simulink model "EECS_419_Homework_4_Speed"  (R2025a)
settings: Solver=VariableStepAuto  StartTime=0.0  StopTime=10.0  RelTol=1e-3
undefined symbols (not defined in the file or in its folder): b_r, H
libraries: slpidlib x3
settings Model: Creator=petercauchy  LastModifiedBy=petercauchy

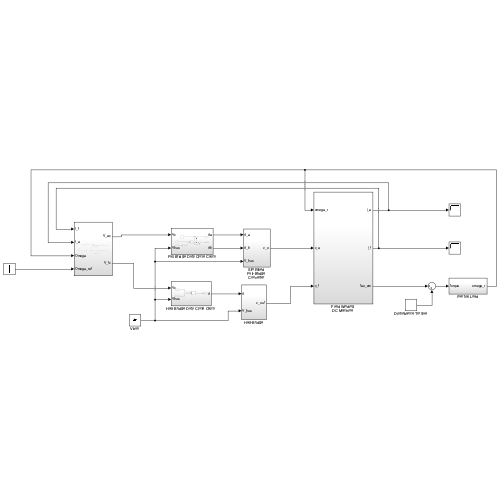
[thumbnail: Simulink's stored preview of the top-level diagram]
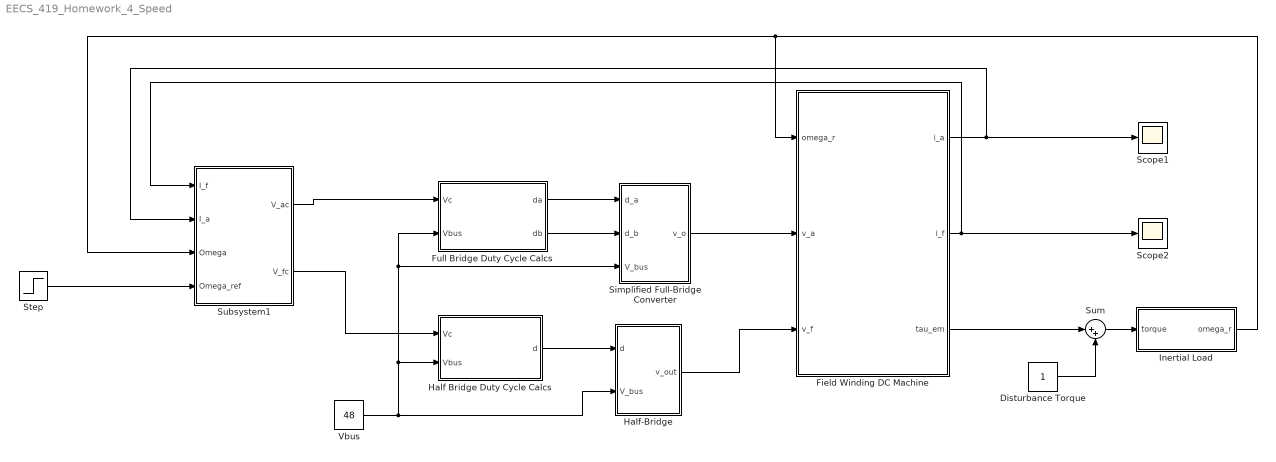
== system EECS_419_Homework_4_Speed ==
  Disturbance Torque : Constant
  Field Winding DC Machine : Subsystem
  Full Bridge Duty Cycle Calcs : Subsystem
  Half Bridge Duty Cycle Calcs : Subsystem
  Half-Bridge : Subsystem
  Inertial Load : Subsystem
  Scope1 : Scope
      settings: ActiveDisplayYMinimum=-27.326179749538095  ActiveDisplayYMaximum=3.1844313093536782
  Scope2 : Scope
      settings: ActiveDisplayYMinimum=-0.0328865701172645  ActiveDisplayYMaximum=0.29597913105538054  DataLoggingVariableName=ScopeData2
  Simplified Full-Bridge Converter : Subsystem
  Step : Step  After=5  SampleTime=0
  Subsystem1 : Subsystem
  Sum : Sum  Inputs=|++
  Vbus : Constant  Value=48
  wires:
  Subsystem1/1(V_ac) -> Full Bridge Duty Cycle Calcs/1(Vc)
  Field Winding DC Machine/3(tau_em) -> Sum/1
  Field Winding DC Machine/1(i_a) -> Scope1/1, Subsystem1/2(I_a)
  Subsystem1/2(V_fc) -> Half Bridge Duty Cycle Calcs/1(Vc)
  Vbus/1 -> Half-Bridge/2(V_bus), Half Bridge Duty Cycle Calcs/2(Vbus), Simplified Full-Bridge Converter/3(V_bus), Full Bridge Duty Cycle Calcs/2(Vbus)
  Half Bridge Duty Cycle Calcs/1(d) -> Half-Bridge/1(d)
  Full Bridge Duty Cycle Calcs/2(db) -> Simplified Full-Bridge Converter/2(d_b)
  Field Winding DC Machine/2(i_f) -> Scope2/1, Subsystem1/1(I_f)
  Full Bridge Duty Cycle Calcs/1(da) -> Simplified Full-Bridge Converter/1(d_a)
  Half-Bridge/1(v_out) -> Field Winding DC Machine/3(v_f)
  Simplified Full-Bridge Converter/1(v_o) -> Field Winding DC Machine/2(v_a)
  Disturbance Torque/1 -> Sum/2
  Sum/1 -> Inertial Load/1(torque)
  Inertial Load/1(omega_r) -> Field Winding DC Machine/1(omega_r), Subsystem1/3(Omega)
  Step/1 -> Subsystem1/4(Omega_ref)

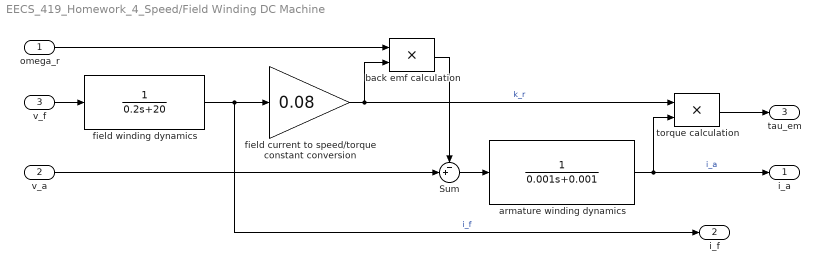
== system EECS_419_Homework_4_Speed/Field Winding DC Machine ==
  omega_r : Inport
  v_a : Inport  Port=2
  v_f : Inport  Port=3
  Sum : Sum  Inputs=-+|  SaturateOnIntegerOverflow=on
  armature winding dynamics : TransferFcn  Denominator=[0.001 0.001]
  back emf calculation : Product  SaturateOnIntegerOverflow=on  OutDataTypeStr=Inherit: Same as first input
  field current to speed/torque constant conversion : Gain  Gain=0.08  SaturateOnIntegerOverflow=on  OutDataTypeStr=Inherit: Same as input  ParamDataTypeStr=Inherit: Same as input
  field winding dynamics : TransferFcn  Denominator=[0.2 20]
  torque calculation : Product  SaturateOnIntegerOverflow=on  OutDataTypeStr=Inherit: Same as first input
  i_a : Outport
  i_f : Outport  Port=2
  tau_em : Outport  Port=3
  wires:
  back emf calculation/1 -> Sum/1
  v_a/1 -> Sum/2
  Sum/1 -> armature winding dynamics/1
  armature winding dynamics/1 -> i_a/1, torque calculation/2  "i_a"
  v_f/1 -> field winding dynamics/1
  field winding dynamics/1 -> i_f/1, field current to speed/torque constant conversion/1  "i_f"
  field current to speed/torque constant conversion/1 -> back emf calculation/2, torque calculation/1  "k_r"
  omega_r/1 -> back emf calculation/1
  torque calculation/1 -> tau_em/1

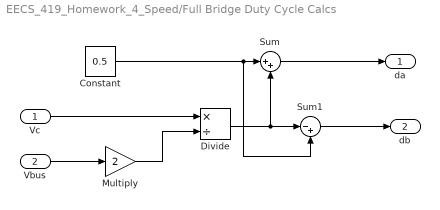
== system EECS_419_Homework_4_Speed/Full Bridge Duty Cycle Calcs ==
  Vc : Inport
  Vbus : Inport  Port=2
  Constant : Constant  Value=0.5
  Divide : Product  Inputs=*/
  Multiply : Gain  Gain=2
  Sum : Sum  Inputs=|++
  Sum1 : Sum  Inputs=|-+
  da : Outport
  db : Outport  Port=2
  wires:
  Vc/1 -> Divide/1
  Vbus/1 -> Multiply/1
  Constant/1 -> Sum1/2, Sum/1
  Sum/1 -> da/1
  Divide/1 -> Sum1/1, Sum/2
  Multiply/1 -> Divide/2
  Sum1/1 -> db/1

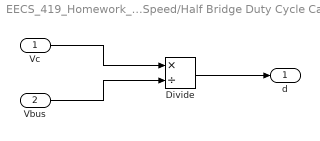
== system EECS_419_Homework_4_Speed/Half Bridge Duty Cycle Calcs ==
  Vc : Inport
  Vbus : Inport  Port=2
  Divide : Product  Inputs=*/
  d : Outport
  wires:
  Vbus/1 -> Divide/2
  Vc/1 -> Divide/1
  Divide/1 -> d/1

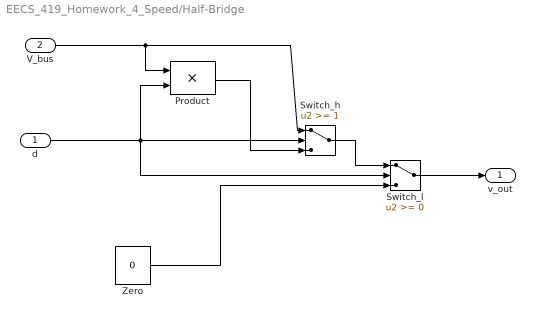
== system EECS_419_Homework_4_Speed/Half-Bridge ==
  d : Inport
  V_bus : Inport  Port=2
  Product : Product  SaturateOnIntegerOverflow=on  OutDataTypeStr=Inherit: Same as first input
  Switch_h : Switch  Threshold=1  InputSameDT=off
  Switch_l : Switch  InputSameDT=off
  Zero : Constant  Value=0
  v_out : Outport  VectorParamsAs1DForOutWhenUnconnected=off
  wires:
  d/1 -> Switch_h/2, Product/2, Switch_l/2
  V_bus/1 -> Switch_h/1, Product/1
  Product/1 -> Switch_h/3
  Zero/1 -> Switch_l/3
  Switch_h/1 -> Switch_l/1
  Switch_l/1 -> v_out/1

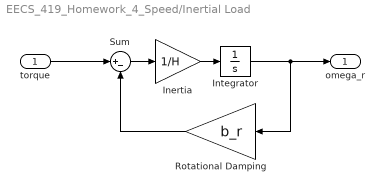
== system EECS_419_Homework_4_Speed/Inertial Load ==
  torque : Inport
  Inertia : Gain  Gain=1/H  SaturateOnIntegerOverflow=on  OutDataTypeStr=Inherit: Same as input  ParamDataTypeStr=Inherit: Same as input
  Integrator : Integrator
  Rotational Damping : Gain  Gain=b_r  SaturateOnIntegerOverflow=on  OutDataTypeStr=Inherit: Same as input  ParamDataTypeStr=Inherit: Same as input
  Sum : Sum  Inputs=|+-  SaturateOnIntegerOverflow=on
  omega_r : Outport
  wires:
  Integrator/1 -> omega_r/1, Rotational Damping/1
  torque/1 -> Sum/1
  Sum/1 -> Inertia/1
  Inertia/1 -> Integrator/1
  Rotational Damping/1 -> Sum/2

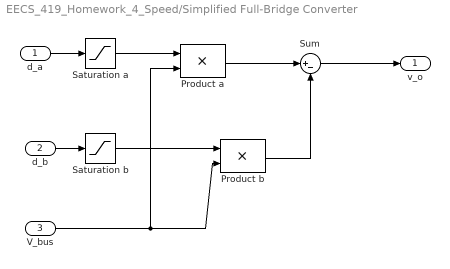
== system EECS_419_Homework_4_Speed/Simplified Full-Bridge Converter ==
  d_a : Inport
  d_b : Inport  Port=2
  V_bus : Inport  Port=3
  Product a : Product  SaturateOnIntegerOverflow=on  OutDataTypeStr=Inherit: Same as first input
  Product b : Product  SaturateOnIntegerOverflow=on  OutDataTypeStr=Inherit: Same as first input
  Saturation a : Saturate  UpperLimit=1  LowerLimit=0
  Saturation b : Saturate  UpperLimit=1  LowerLimit=0
  Sum : Sum  Inputs=|+-  SaturateOnIntegerOverflow=on
  v_o : Outport  VectorParamsAs1DForOutWhenUnconnected=off
  wires:
  d_a/1 -> Saturation a/1
  d_b/1 -> Saturation b/1
  Product a/1 -> Sum/1
  Product b/1 -> Sum/2
  Sum/1 -> v_o/1
  Saturation a/1 -> Product a/1
  V_bus/1 -> Product a/2, Product b/2
  Saturation b/1 -> Product b/1

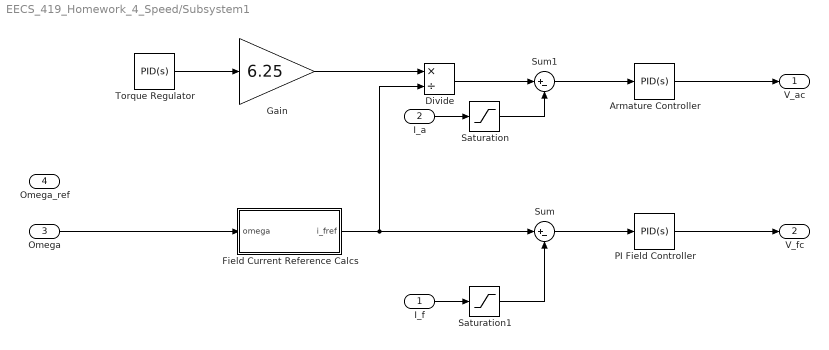
== system EECS_419_Homework_4_Speed/Subsystem1 ==
  I_f : Inport
  I_a : Inport  Port=2
  Omega : Inport  Port=3
  Omega_ref : Inport  Port=4
  Armature Controller : slpidlib/PID Controller  Controller=PID  Form=Parallel  TimeDomain=Continuous-time  UseExternalTs=off  SampleTime=-1  IntegratorMethod=Forward Euler  FilterMethod=Forward Euler  ControllerParametersSource=internal  P=6.28  I=6.28  UseKiTs=off  D=0  UseExternalDerivativeSource=off  N=1  UseFilter=on  TunerSelectOption=Transfer Function Based (PID Tuner App)  InitialConditionSource=internal  InitialConditionForIntegrator=0  InitialConditionForFilter=0  DifferentiatorICPrevScaledInput=0  ExternalReset=none  TrackingMode=off  Kt=1  LimitOutput=on  SatLimitsSource=internal  UpperSaturationLimit=48  LowerSaturationLimit=-48  LinearizeAsGain=on  AntiWindupMode=none  Kb=1  LimitIntegrator=off  UpperIntegratorSaturationLimit=inf  LowerIntegratorSaturationLimit=-inf  POutMin=[]  POutMax=[]  IOutMin=[]  IOutMax=[]  DOutMin=[]  DOutMax=[]  NOutMin=[]  NOutMax=[]  SumOutMin=[]  SumOutMax=[]  SaturationOutMin=[]  SaturationOutMax=[]  PParamMin=[]  PParamMax=[]  IParamMin=[]  IParamMax=[]  DParamMin=[]  DParamMax=[]  NParamMin=[]  NParamMax=[]  KbParamMin=[]  KbParamMax=[]  KtParamMin=[]  KtParamMax=[]  KbOutMin=[]  KbOutMax=[]  KtOutMin=[]  KtOutMax=[]  IntegratorOutMin=[]  IntegratorOutMax=[]  FilterOutMin=[]  FilterOutMax=[]  SumI1OutMin=[]  SumI1OutMax=[]  SumI2OutMin=[]  SumI2OutMax=[]  SumI3OutMin=[]  SumI3OutMax=[]  SumI4OutMin=[]  SumI4OutMax=[]  SumDOutMin=[]  SumDOutMax=[]  DifferentiatorOutMin=[]  DifferentiatorOutMax=[]  FilterDiffOutCoefMin=[]  FilterDiffOutCoefMax=[]  ReciprocalOutMin=[]  ReciprocalOutMax=[]  SumDenOutMin=[]  SumDenOutMax=[]  SumNumOutMin=[]  SumNumOutMax=[]  DivideOutMin=[]  DivideOutMax=[]  UdiffTsProdOutMin=[]  UdiffTsProdOutMax=[]  NTsProdOutMin=[]  NTsProdOutMax=[]  UintegralTsProdOutMin=[]  UintegralTsProdOutMax=[]  UngainTsProdOutMin=[]  UngainTsProdOutMax=[]  ClampingZeroOutDataTypeStr=Inherit: Inherit via back propagation  ClampingZeroOutMin=[]  ClampingZeroOutMax=[]  FilterDenConstantOutDataTypeStr=Inherit: Inherit via back propagation  FilterDenConstantOutMin=[]  FilterDenConstantOutMax=[]  PCopyOutDataTypeStr=Inherit: Inherit via back propagation  PCopyOutMin=[]  PCopyOutMax=[]  NCopyOutDataTypeStr=Inherit: Inherit via back propagation  NCopyOutMin=[]  NCopyOutMax=[]  IntegratorContinuousStateAttributes=''  IntegratorStateMustResolveToSignalObject=off  IntegratorRTWStateStorageClass=Auto  FilterContinuousStateAttributes=''  FilterStateMustResolveToSignalObject=off  FilterRTWStateStorageClass=Auto  ParallelPVariant=InternalParameters  IdealPVariant=Disabled  IVariant=InternalParameters  DVariant=InternalParameters  IntegratorVariant=Continuous  SatVariant=Enabled  AWVariant=Passthrough  PCopyVariant=Disabled  TRVariant=Disabled  FdbkBlocksVariant=Forward  IdealPFdbkVariant=Disabled  SatFdbkVariant=Disabled  DerivativeFilterVariant=ContFilter  NVariant=InternalParameters  NCopyVariant=Disabled  FilterICVariant=InternalICsFilter  IntegratorICVariant=InternalICs  ExternalResetVariant=Disabled  TRSumVariant=Passthrough  SumFdbkVariant=Disabled  SumVariant=Sum_PID  TsampFilterVariant=InternalTs  TsampNgainVariant=Passthrough  TsampIntegralVariant=Disabled_SignalSpec  ExternalSaturationOutDataTypeStr=Inherit: Same as second input  DerivativeSourceVariant=ErrorSignal  PreIntVariant=InternalPreInt
  Divide : Product  Inputs=*/
  Field Current Reference Calcs : Subsystem
  Gain : Gain  Gain=6.25
  PI Field Controller : slpidlib/PID Controller  Controller=PID  Form=Parallel  TimeDomain=Continuous-time  UseExternalTs=off  SampleTime=-1  IntegratorMethod=Forward Euler  FilterMethod=Forward Euler  ControllerParametersSource=internal  P=1256.6  I=1.256e6  UseKiTs=off  D=0  UseExternalDerivativeSource=off  N=1  UseFilter=on  TunerSelectOption=Transfer Function Based (PID Tuner App)  InitialConditionSource=internal  InitialConditionForIntegrator=0  InitialConditionForFilter=0  DifferentiatorICPrevScaledInput=0  ExternalReset=none  TrackingMode=off  Kt=1  LimitOutput=on  SatLimitsSource=internal  UpperSaturationLimit=48  LowerSaturationLimit=0  LinearizeAsGain=on  AntiWindupMode=none  Kb=1  LimitIntegrator=off  UpperIntegratorSaturationLimit=inf  LowerIntegratorSaturationLimit=-inf  POutMin=[]  POutMax=[]  IOutMin=[]  IOutMax=[]  DOutMin=[]  DOutMax=[]  NOutMin=[]  NOutMax=[]  SumOutMin=[]  SumOutMax=[]  SaturationOutMin=[]  SaturationOutMax=[]  PParamMin=[]  PParamMax=[]  IParamMin=[]  IParamMax=[]  DParamMin=[]  DParamMax=[]  NParamMin=[]  NParamMax=[]  KbParamMin=[]  KbParamMax=[]  KtParamMin=[]  KtParamMax=[]  KbOutMin=[]  KbOutMax=[]  KtOutMin=[]  KtOutMax=[]  IntegratorOutMin=[]  IntegratorOutMax=[]  FilterOutMin=[]  FilterOutMax=[]  SumI1OutMin=[]  SumI1OutMax=[]  SumI2OutMin=[]  SumI2OutMax=[]  SumI3OutMin=[]  SumI3OutMax=[]  SumI4OutMin=[]  SumI4OutMax=[]  SumDOutMin=[]  SumDOutMax=[]  DifferentiatorOutMin=[]  DifferentiatorOutMax=[]  FilterDiffOutCoefMin=[]  FilterDiffOutCoefMax=[]  ReciprocalOutMin=[]  ReciprocalOutMax=[]  SumDenOutMin=[]  SumDenOutMax=[]  SumNumOutMin=[]  SumNumOutMax=[]  DivideOutMin=[]  DivideOutMax=[]  UdiffTsProdOutMin=[]  UdiffTsProdOutMax=[]  NTsProdOutMin=[]  NTsProdOutMax=[]  UintegralTsProdOutMin=[]  UintegralTsProdOutMax=[]  UngainTsProdOutMin=[]  UngainTsProdOutMax=[]  ClampingZeroOutDataTypeStr=Inherit: Inherit via back propagation  ClampingZeroOutMin=[]  ClampingZeroOutMax=[]  FilterDenConstantOutDataTypeStr=Inherit: Inherit via back propagation  FilterDenConstantOutMin=[]  FilterDenConstantOutMax=[]  PCopyOutDataTypeStr=Inherit: Inherit via back propagation  PCopyOutMin=[]  PCopyOutMax=[]  NCopyOutDataTypeStr=Inherit: Inherit via back propagation  NCopyOutMin=[]  NCopyOutMax=[]  IntegratorContinuousStateAttributes=''  IntegratorStateMustResolveToSignalObject=off  IntegratorRTWStateStorageClass=Auto  FilterContinuousStateAttributes=''  FilterStateMustResolveToSignalObject=off  FilterRTWStateStorageClass=Auto  ParallelPVariant=InternalParameters  IdealPVariant=Disabled  IVariant=InternalParameters  DVariant=InternalParameters  IntegratorVariant=Continuous  SatVariant=Enabled  AWVariant=Passthrough  PCopyVariant=Disabled  TRVariant=Disabled  FdbkBlocksVariant=Forward  IdealPFdbkVariant=Disabled  SatFdbkVariant=Disabled  DerivativeFilterVariant=ContFilter  NVariant=InternalParameters  NCopyVariant=Disabled  FilterICVariant=InternalICsFilter  IntegratorICVariant=InternalICs  ExternalResetVariant=Disabled  TRSumVariant=Passthrough  SumFdbkVariant=Disabled  SumVariant=Sum_PID  TsampFilterVariant=InternalTs  TsampNgainVariant=Passthrough  TsampIntegralVariant=Disabled_SignalSpec  ExternalSaturationOutDataTypeStr=Inherit: Same as second input  DerivativeSourceVariant=ErrorSignal  PreIntVariant=InternalPreInt
  Saturation : Saturate  UpperLimit=100  LowerLimit=-100
  Saturation1 : Saturate  UpperLimit=1  LowerLimit=-1
  Sum : Sum  Inputs=|+-
  Sum1 : Sum  Inputs=|+-
  Torque Regulator : slpidlib/PID Controller  Controller=PID  Form=Parallel  TimeDomain=Continuous-time  UseExternalTs=off  SampleTime=-1  IntegratorMethod=Forward Euler  FilterMethod=Forward Euler  ControllerParametersSource=internal  P=78.5  I=78.5  UseKiTs=off  D=0  UseExternalDerivativeSource=off  N=1  UseFilter=on  TunerSelectOption=Transfer Function Based (PID Tuner App)  InitialConditionSource=internal  InitialConditionForIntegrator=0  InitialConditionForFilter=0  DifferentiatorICPrevScaledInput=0  ExternalReset=none  TrackingMode=off  Kt=1  LimitOutput=off  SatLimitsSource=internal  UpperSaturationLimit=inf  LowerSaturationLimit=-inf  LinearizeAsGain=on  AntiWindupMode=none  Kb=1  LimitIntegrator=off  UpperIntegratorSaturationLimit=inf  LowerIntegratorSaturationLimit=-inf  POutMin=[]  POutMax=[]  IOutMin=[]  IOutMax=[]  DOutMin=[]  DOutMax=[]  NOutMin=[]  NOutMax=[]  SumOutMin=[]  SumOutMax=[]  SaturationOutMin=[]  SaturationOutMax=[]  PParamMin=[]  PParamMax=[]  IParamMin=[]  IParamMax=[]  DParamMin=[]  DParamMax=[]  NParamMin=[]  NParamMax=[]  KbParamMin=[]  KbParamMax=[]  KtParamMin=[]  KtParamMax=[]  KbOutMin=[]  KbOutMax=[]  KtOutMin=[]  KtOutMax=[]  IntegratorOutMin=[]  IntegratorOutMax=[]  FilterOutMin=[]  FilterOutMax=[]  SumI1OutMin=[]  SumI1OutMax=[]  SumI2OutMin=[]  SumI2OutMax=[]  SumI3OutMin=[]  SumI3OutMax=[]  SumI4OutMin=[]  SumI4OutMax=[]  SumDOutMin=[]  SumDOutMax=[]  DifferentiatorOutMin=[]  DifferentiatorOutMax=[]  FilterDiffOutCoefMin=[]  FilterDiffOutCoefMax=[]  ReciprocalOutMin=[]  ReciprocalOutMax=[]  SumDenOutMin=[]  SumDenOutMax=[]  SumNumOutMin=[]  SumNumOutMax=[]  DivideOutMin=[]  DivideOutMax=[]  UdiffTsProdOutMin=[]  UdiffTsProdOutMax=[]  NTsProdOutMin=[]  NTsProdOutMax=[]  UintegralTsProdOutMin=[]  UintegralTsProdOutMax=[]  UngainTsProdOutMin=[]  UngainTsProdOutMax=[]  ClampingZeroOutDataTypeStr=Inherit: Inherit via back propagation  ClampingZeroOutMin=[]  ClampingZeroOutMax=[]  FilterDenConstantOutDataTypeStr=Inherit: Inherit via back propagation  FilterDenConstantOutMin=[]  FilterDenConstantOutMax=[]  PCopyOutDataTypeStr=Inherit: Inherit via back propagation  PCopyOutMin=[]  PCopyOutMax=[]  NCopyOutDataTypeStr=Inherit: Inherit via back propagation  NCopyOutMin=[]  NCopyOutMax=[]  IntegratorContinuousStateAttributes=''  IntegratorStateMustResolveToSignalObject=off  IntegratorRTWStateStorageClass=Auto  FilterContinuousStateAttributes=''  FilterStateMustResolveToSignalObject=off  FilterRTWStateStorageClass=Auto  ParallelPVariant=InternalParameters  IdealPVariant=Disabled  IVariant=InternalParameters  DVariant=InternalParameters  IntegratorVariant=Continuous  SatVariant=Disabled  AWVariant=Passthrough  PCopyVariant=Disabled  TRVariant=Disabled  FdbkBlocksVariant=Forward  IdealPFdbkVariant=Disabled  SatFdbkVariant=Disabled  DerivativeFilterVariant=ContFilter  NVariant=InternalParameters  NCopyVariant=Disabled  FilterICVariant=InternalICsFilter  IntegratorICVariant=InternalICs  ExternalResetVariant=Disabled  TRSumVariant=Passthrough  SumFdbkVariant=Disabled  SumVariant=Sum_PID  TsampFilterVariant=InternalTs  TsampNgainVariant=Passthrough  TsampIntegralVariant=Disabled_SignalSpec  ExternalSaturationOutDataTypeStr=Inherit: Same as second input  DerivativeSourceVariant=ErrorSignal  PreIntVariant=InternalPreInt
  V_ac : Outport
  V_fc : Outport  Port=2
  wires:
  PI Field Controller/1 -> V_fc/1
  I_f/1 -> Saturation1/1
  Sum/1 -> PI Field Controller/1
  Field Current Reference Calcs/1(i_fref) -> Divide/2, Sum/1
  Omega/1 -> Field Current Reference Calcs/1(omega)
  Armature Controller/1 -> V_ac/1
  Sum1/1 -> Armature Controller/1
  Divide/1 -> Sum1/1
  Torque Regulator/1 -> Gain/1
  Gain/1 -> Divide/1
  I_a/1 -> Saturation/1
  Saturation/1 -> Sum1/2
  Saturation1/1 -> Sum/2

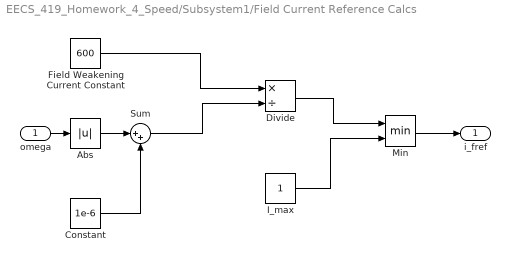
== system EECS_419_Homework_4_Speed/Subsystem1/Field Current Reference Calcs ==
  omega : Inport
  Abs : Abs  SaturateOnIntegerOverflow=off
  Constant : Constant  Value=1e-6
  Divide : Product  Inputs=*/
  Field Weakening Current Constant : Constant  Value=600
  I_max : Constant
  Min : MinMax  Inputs=2
  Sum : Sum  Inputs=|++
  i_fref : Outport
  wires:
  omega/1 -> Abs/1
  Field Weakening Current Constant/1 -> Divide/1
  Min/1 -> i_fref/1
  I_max/1 -> Min/2
  Divide/1 -> Min/1
  Abs/1 -> Sum/1
  Constant/1 -> Sum/2
  Sum/1 -> Divide/2
